simulink model "PEDPROJECTREAL_V3_fixed_2"  (R2026a)
settings: Solver=ode23t  StopTime=5  MaxStep=1e-4
libraries: fl_lib x20, nesl_utility x12, ee_lib x7
(part 2 of 2)

== matlab function PEDPROJECTREAL_V3_fixed_2/STM32_Controller ==
  data: Target_RPM input; PWM_Pulses output; Va input; Vb input; Vc input
function PWM_Pulses = stm32_controller(Target_RPM, Va, Vb, Vc)
    persistent hall_state pwm_cnt;
    if isempty(hall_state)
        hall_state = uint8(1); pwm_cnt = 0;
    end
    pwm_cnt = pwm_cnt + 1;
    if pwm_cnt > 100, pwm_cnt = 0; end
    threshold = 0.5;
    if Va > threshold && Vb < -threshold, hall_state = uint8(1);
    elseif Va > threshold && Vc < -threshold, hall_state = uint8(2);
    elseif Vb > threshold && Vc < -threshold, hall_state = uint8(3);
    elseif Vb > threshold && Va < -threshold, hall_state = uint8(4);
    elseif Vc > threshold && Va < -threshold, hall_state = uint8(5);
    elseif Vc > threshold && Vb < -threshold, hall_state = uint8(6); end
    duty = max(0, min(100, Target_RPM / 50));
    pwm = (pwm_cnt < duty);
    switch hall_state
        case 1, PWM_Pulses = [pwm 0 0 0 0 1];
        case 2, PWM_Pulses = [pwm 0 0 1 0 0];
        case 3, PWM_Pulses = [0 0 pwm 0 0 0];
        case 4, PWM_Pulses = [0 1 pwm 0 0 0];
        case 5, PWM_Pulses = [0 0 0 0 pwm 0];
        case 6, PWM_Pulses = [0 0 0 0 pwm 1];
        otherwise, PWM_Pulses = zeros(1, 6);
    end
